simulink library "FAM_lab_scale_v4"  (R2024a)
settings: Solver=VariableStepAuto  StartTime=0.0  StopTime=10.0  RelTol=1e-3
undefined symbols (not defined in the file): FAM_elasticity, FAM_stretched_radius, FAM_unstretched_length, FAM_wall_thickness, fiber_angle_alpha, fiber_angle_alpha_unstr, hose_pump_force_enabled, hose_pump_max_stretch, hose_pump_throughFlow_adjust
settings Model: Creator=cmmcguir  LastModifiedBy=Carson
settings RTWCC: GPUComputeCapability=3.5

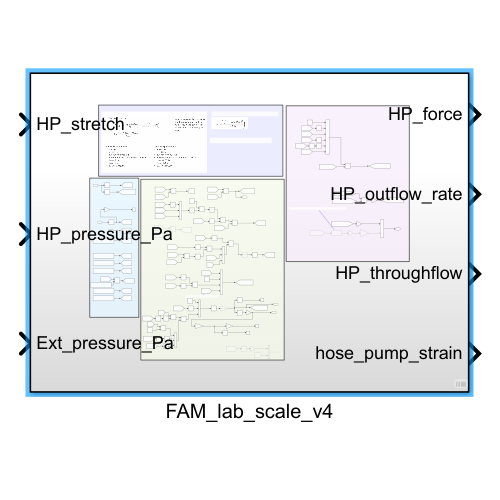
[thumbnail: Simulink's stored preview of the top-level diagram]
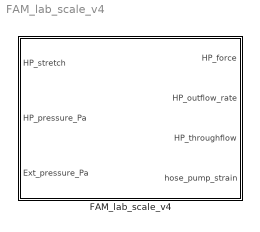
== system FAM_lab_scale_v4 ==
  FAM_lab_scale_v4 : Subsystem

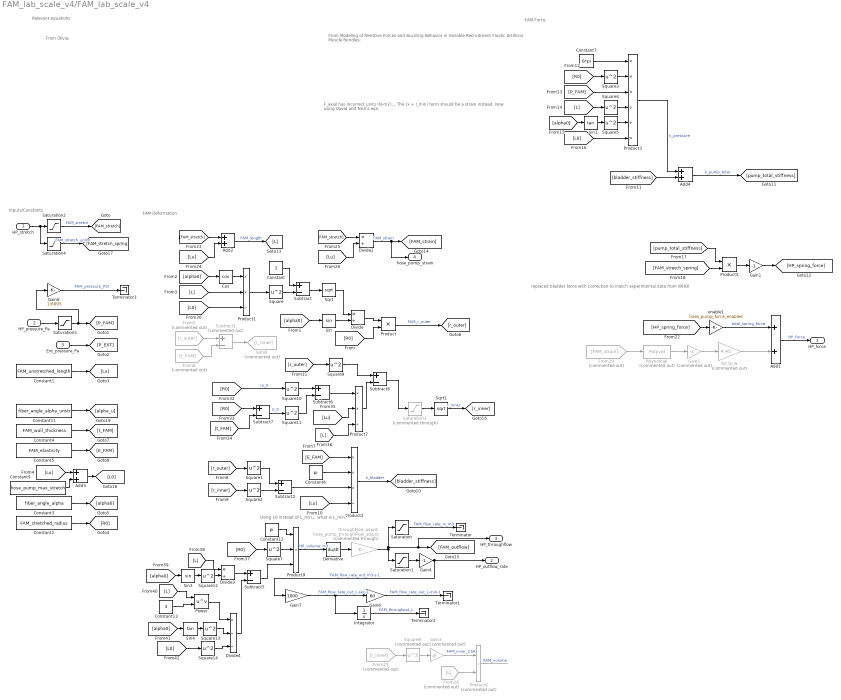
== system FAM_lab_scale_v4/FAM_lab_scale_v4 ==
  note: replaced bladder force with correction to match experimental data from WHOI
  note: F_axial has incorrect units (N-m2)... The (x + l_min) term should be a strain instead. Now using David and Nick's eqn.
  note: FAM Force
  note: FAM Deformation
  note: Inputs/Constants
  note: Relevant equations
  note: From Modeling of Resistive Forces and Buckling Behavior in Variable Recruitment Fluidic Artificial Muscle Bundles:
  note: From Olivia:
  note: Using L0 instead of L_min... what is L_min?
  HP_stretch : Inport  Unit=m
  HP_pressure_Pa : Inport  Port=2  Unit=Pa
  Ext_pressure_Pa : Inport  Port=3  Unit=Pa
  Add{1..4} (4 alike) : Sum
  Constant : Constant
  Constant1 : Constant  Value=FAM_unstretched_length
  Constant11 : Constant  Value=fiber_angle_alpha_unstr
  Constant12 : Constant  Value=pi
  Constant13 : Constant  Value=3
  Constant2 : Constant  Value=FAM_stretched_radius
  Constant3 : Constant  Value=fiber_angle_alpha
  Constant4 : Constant  Value=FAM_wall_thickness
  Constant5 : Constant  Value=FAM_elasticity
  Constant6 : Constant  Value=pi
  Constant7 : Constant  Value=6*pi
  Constant9 : Constant  Value=hose_pump_max_stretch
  Cos : Trigonometry  Operator=cos
  Derivative : Derivative
  Divide : Product  Inputs=*/
  Divide2 : Product  Inputs=*/
  Divide3 : Product  Inputs=*/
  Divide4 : Product  Inputs=*//
  From27 : From  Commented=on  GotoTag=r_inner
  From28 : From  Commented=on  GotoTag=L
  From29 : From  Commented=on  GotoTag=FAM_strain
  From5 : From  Commented=on  GotoTag=r_outer
  From6 : From  Commented=on  GotoTag=t_FAM
  Gain1 : Gain  Gain=-1
  Gain3 : Gain  Commented=on  Gain=pi
  Gain4 : Gain  Gain=-1
  Gain5 : Gain  Commented=on  Gain=-1
  Gain6 : Gain  Gain=60
  Gain7 : Gain  Gain=1000
  Gain8 : Gain  Gain=1/6895
  Goto8 : Goto  Commented=on  GotoTag=r_inner
  Integrator : Integrator
  Polynomial : Polyval  Commented=on  Coefs="1e5* [1.5724   -0.4144    0.0729   -0.0014]"
  Power : Math  Operator=pow
  Product : Product
  Product1 : Product  Inputs=**/
  Product2 : Product  Inputs=***/
  Product3 : Product  Inputs=***//*
  Product5 : Product
  Product6 : Product  Commented=on
  Product7 : Product  Inputs=**/
  Product9 : Product  Inputs=***
  Saturation : Saturate  UpperLimit=inf  LowerLimit=0  ZeroCross=off
  Saturation1 : Saturate  UpperLimit=0  LowerLimit=-inf  ZeroCross=off
  Saturation2 : Saturate  UpperLimit=hose_pump_max_stretch  LowerLimit=0
  Saturation3 : Saturate  Commented=through  UpperLimit=inf  LowerLimit=(FAM_wall_thickness*1.1)^2
  Saturation4 : Saturate  UpperLimit=inf  LowerLimit=0
  Saturation5 : Saturate  UpperLimit=inf  LowerLimit=0
  Sin : Trigonometry
  Sin1 : Trigonometry  Operator=tan
  Sin3 : Trigonometry
  Sin4 : Trigonometry  Operator=tan
  Sqrt : Sqrt
  Sqrt1 : Sqrt
  Square{,1..5,7,9..14} (13 alike) : Math  Operator=square
  Square8 : Math  Commented=on  Operator=square
  Subtract{,2,5..8} (6 alike) : Sum  Inputs=+-
  Subtract1 : Sum  Commented=on  Inputs=+-
  Terminator{,1..3} (4 alike) : Terminator
  enable1 : Gain  Gain=hose_pump_force_enabled
  lbf_to_N : Gain  Commented=on  Gain=4.45
  throughFlow_adjust : Gain  Commented=through  Gain=hose_pump_throughFlow_adjust
  HP_force : Outport
  HP_outflow_rate : Outport  Port=2
  HP_throughflow : Outport  Port=3
  hose_pump_strain : Outport  Port=4
  wires:
  [FAM_stretch_spring] -> Product5/2
  [E_FAM] -> Product2/1
  Constant3/1 -> [alpha0]
  [R0] -> Product/2
  Product2/1 -> [bladder_stiffness]  "k_bladder"
  From6/1 -> Subtract1/2
  Constant2/1 -> [R0]
  Ext_pressure_Pa/1 -> [P_EXT]
  [alpha0] -> Cos/1
  [pump_total_stiffness] -> Product5/1
  Subtract2/1 -> Product2/3
  Product/1 -> [r_outer]  "FAM_r_outer"
  Product5/1 -> Gain1/1
  Constant4/1 -> [t_FAM]
  Cos/1 -> Product1/1
  HP_pressure_Pa/1 -> Saturation5/1
  Subtract/1 -> Sqrt/1
  [HP_spring_force] -> enable1/1
  Constant/1 -> Subtract/1
  [Lu] -> Product2/4
  Add1/1 -> HP_force/1  "HP_force"
  [r_outer] -> Square1/1
  Constant1/1 -> [Lu]
  Square/1 -> Subtract/2
  Constant6/1 -> Product2/2
  Divide/1 -> Product/1
  From5/1 -> Subtract1/1
  Subtract1/1 -> Goto8/1
  Sqrt/1 -> Divide/1
  [L] -> Product1/2
  Square1/1 -> Subtract2/1
  Product1/1 -> Square/1
  Constant5/1 -> [E_FAM]
  Square2/1 -> Subtract2/2
  Sin/1 -> Divide/2
  [alpha0] -> Sin/1
  [r_inner] -> Square2/1
  [FAM_stretch] -> Add2/1
  [Lu] -> Add2/2
  Add2/1 -> [L]  "FAM_length"
  Divide2/1 -> hose_pump_strain/1, [FAM_strain]  "FAM_strain"
  [Lu] -> Divide2/2
  [FAM_stretch] -> Divide2/1
  Gain1/1 -> [HP_spring_force]
  Derivative/1 -> throughFlow_adjust/1
  Saturation/1 -> Terminator/1  "FAM_flow_rate_in_m3"
  Gain4/1 -> HP_outflow_rate/1, Gain7/1  "FAM_flow_rate_out_m3-s-1"
  Saturation1/1 -> Gain4/1
  Gain6/1 -> Terminator1/1  "FAM_flow_rate_out_L-min-1"
  Gain7/1 -> Integrator/1, Gain6/1  "FAM_flow_rate_out_L-sec-1"
  Integrator/1 -> Terminator2/1  "FAM_throughput_L"
  Saturation2/1 -> [FAM_stretch]  "FAM_stretch"
  [r_outer] -> Square9/1
  [R0] -> Square10/1  "ro_0"
  Square10/1 -> Subtract6/1
  [R0] -> Subtract7/1
  [t_FAM] -> Subtract7/2
  Subtract7/1 -> Square11/1  "ri_0"
  Square11/1 -> Subtract6/2
  Subtract6/1 -> Product7/1
  [Lu] -> Product7/2
  Subtract8/1 -> Saturation3/1
  [L] -> Product7/3
  From29/1 -> Polynomial/1
  Polynomial/1 -> Gain5/1
  Gain5/1 -> lbf_to_N/1
  lbf_to_N/1 -> Add1/2
  Square9/1 -> Subtract8/1
  Product7/1 -> Subtract8/2
  HP_stretch/1 -> Saturation4/1, Saturation2/1
  Sqrt1/1 -> [r_inner]  "r_inner"
  Saturation3/1 -> Sqrt1/1
  Saturation4/1 -> [FAM_stretch_spring]  "FAM_stretch_unlim"
  Saturation5/1 -> Gain8/1, [P_FAM]
  Gain8/1 -> Terminator3/1  "FAM_pressure_PSI"
  throughFlow_adjust/1 -> Saturation1/1, Saturation/1, HP_throughflow/1, [FAM_outflow]
  enable1/1 -> Add1/1  "total_spring_force"
  Constant9/1 -> Add3/2
  [Lu] -> Add3/1
  Add3/1 -> [L0]
  Constant11/1 -> [alpha_u]
  [L0] -> Product1/3
  Product6/1 -> ?  "FAM_volume"
  From27/1 -> Square8/1
  Square8/1 -> Gain3/1
  Gain3/1 -> Product6/1  "FAM_inner_CSA"
  From28/1 -> Product6/2
  Product9/1 -> Derivative/1  "HP_volume_m3"
  Constant12/1 -> Product9/1
  [R0] -> Square7/1
  Square7/1 -> Product9/2
  Subtract5/1 -> Product9/3
  Divide3/1 -> Subtract5/1
  Divide4/1 -> Subtract5/2
  [L] -> Divide3/1
  [alpha0] -> Sin3/1
  Square12/1 -> Divide3/2
  Sin3/1 -> Square12/1
  Sin4/1 -> Square13/1
  [alpha0] -> Sin4/1
  [L] -> Power/1
  Power/1 -> Divide4/1
  Square13/1 -> Divide4/2
  Constant13/1 -> Power/2
  [L0] -> Square14/1
  Square14/1 -> Divide4/3
  [bladder_stiffness] -> Add4/2
  Add4/1 -> [pump_total_stiffness]  "k_pump_total"
  Product3/1 -> Add4/1  "k_pressure"
  Constant7/1 -> Product3/1
  [R0] -> Square3/1
  Square3/1 -> Product3/2
  [P_FAM] -> Product3/3
  [L] -> Square4/1
  Square4/1 -> Product3/4
  Sin1/1 -> Square5/1
  [alpha0] -> Sin1/1
  Square5/1 -> Product3/5
  [L0] -> Product3/6
